simulink model "PX4OutputMappingQuadrotor"  (R2026a)
settings: Solver=ode4  FixedStep=stepSize_s
undefined symbols (not defined in the file): MotorCommandHexBus
settings Model: Creator=Edison Altamirano  LastModifiedBy=Edison Altamirano

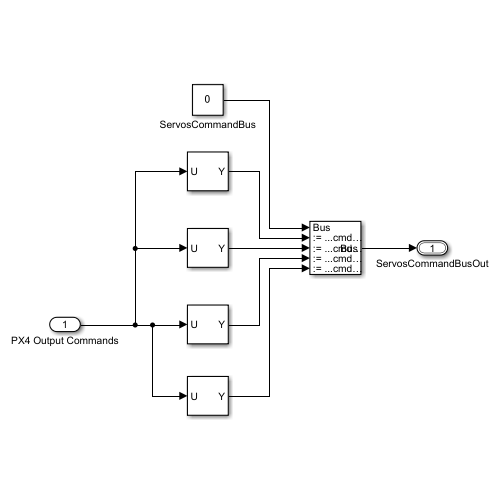
[thumbnail: Simulink's stored preview of the top-level diagram]
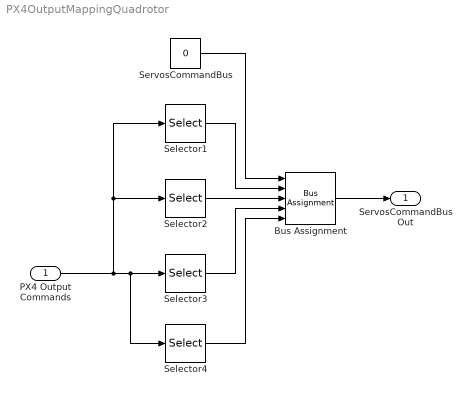
== system PX4OutputMappingQuadrotor ==
  PX4 Output Commands : Inport  PortDimensions=16
  Bus Assignment : BusAssignment  AssignedSignals=MotorCommandHexBus.cmdRotor1_nd,MotorCommandHexBus.cmdRotor2_nd,MotorCommandHexBus.cmdRotor3_nd,MotorCommandHexBus.cmdRotor4_nd
  Selector1 : Selector  InputPortWidth=16  IndexOptions=Index vector (dialog)  Indices=1  OutputSizes=1
  Selector2 : Selector  InputPortWidth=16  IndexOptions=Index vector (dialog)  Indices=2  OutputSizes=1
  Selector3 : Selector  InputPortWidth=16  IndexOptions=Index vector (dialog)  Indices=3  OutputSizes=1
  Selector4 : Selector  InputPortWidth=16  IndexOptions=Index vector (dialog)  Indices=4  OutputSizes=1
  ServosCommandBus : Constant  Value=0  OutDataTypeStr=Bus: ServosCommandBus
  ServosCommandBusOut : Outport  OutDataTypeStr=Bus: ServosCommandBus
  wires:
  Bus Assignment/1 -> ServosCommandBusOut/1
  Selector4/1 -> Bus Assignment/5
  Selector3/1 -> Bus Assignment/4
  Selector2/1 -> Bus Assignment/3
  Selector1/1 -> Bus Assignment/2
  ServosCommandBus/1 -> Bus Assignment/1
  PX4 Output Commands/1 -> Selector3/1, Selector4/1, Selector1/1, Selector2/1
